simulink model "battery_subsystem"  (R2015a)
settings: Solver=ode23t  StartTime=0.0  StopTime=100  RelTol=1e-3  AbsTol=1e-3
libraries: fl_lib x96
settings Model: CovSFcnEnable=off  Creator=jrivitus  LastModifiedBy=sseshadr
settings OptimizationCC: ExpressionDepthLimit=2147483647
settings DebuggingCC: UnderspecifiedInitializationDetection=Classic  MergeDetectMultiDrivingBlocksExec=none  ParameterPrecisionLossMsg=none  FcnCallInpInsideContextMsg=UseLocalSettings  StateNameClashWarn=warning
settings GRTTargetCC: CombineOutputUpdateFcns=off  GRTInterface=on

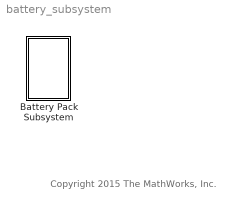
== system battery_subsystem ==
  note: Copyright 2015 The MathWorks, Inc.
  Battery Pack Subsystem : Subsystem

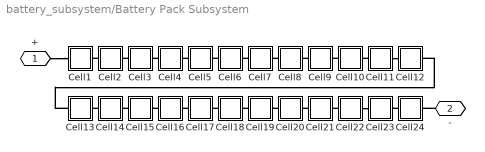
== system battery_subsystem/Battery Pack Subsystem ==
  Cell1 : Subsystem
  Cell10 : Subsystem
  Cell11 : Subsystem
  Cell12 : Subsystem
  Cell13 : Subsystem
  Cell14 : Subsystem
  Cell15 : Subsystem
  Cell16 : Subsystem
  Cell17 : Subsystem
  Cell18 : Subsystem
  Cell19 : Subsystem
  Cell2 : Subsystem
  Cell20 : Subsystem
  Cell21 : Subsystem
  Cell22 : Subsystem
  Cell23 : Subsystem
  Cell24 : Subsystem
  Cell3 : Subsystem
  Cell4 : Subsystem
  Cell5 : Subsystem
  Cell6 : Subsystem
  Cell7 : Subsystem
  Cell8 : Subsystem
  Cell9 : Subsystem
  + : PMIOPort  Port=1  Side=Right
  - : PMIOPort  Port=2  Side=Right
  connections:
  +/RConn1 -- Cell1/LConn1
  Cell2/LConn1 -- Cell1/RConn1
  Cell3/LConn1 -- Cell2/RConn1
  Cell4/LConn1 -- Cell3/RConn1
  Cell5/LConn1 -- Cell4/RConn1
  Cell6/LConn1 -- Cell5/RConn1
  Cell7/LConn1 -- Cell6/RConn1
  Cell8/LConn1 -- Cell7/RConn1
  Cell9/LConn1 -- Cell8/RConn1
  Cell10/LConn1 -- Cell9/RConn1
  Cell11/LConn1 -- Cell10/RConn1
  Cell13/LConn1 -- Cell12/RConn1
  Cell14/LConn1 -- Cell13/RConn1
  Cell15/LConn1 -- Cell14/RConn1
  Cell16/LConn1 -- Cell15/RConn1
  Cell17/LConn1 -- Cell16/RConn1
  Cell18/LConn1 -- Cell17/RConn1
  Cell19/LConn1 -- Cell18/RConn1
  Cell20/LConn1 -- Cell19/RConn1
  Cell21/LConn1 -- Cell20/RConn1
  Cell22/LConn1 -- Cell21/RConn1
  Cell24/LConn1 -- Cell23/RConn1
  -/RConn1 -- Cell24/RConn1
  Cell11/RConn1 -- Cell12/LConn1
  Cell22/RConn1 -- Cell23/LConn1

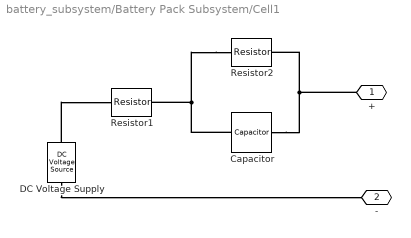
== system battery_subsystem/Battery Pack Subsystem/Cell1 ==
  Capacitor : fl_lib/Electrical/Electrical Elements/Capacitor  c=1e-3 F  r=1e-6 Ohm  g=0 1/Ohm  i_specify=off  i_priority=High  i=0 A  v_specify=off  v_priority=High  v=0 V  vc_specify=on  vc_priority=High  vc=0 V
  DC Voltage Supply : fl_lib/Electrical/Electrical Sources/DC Voltage Source  v0=4.2 V
  Resistor1 : fl_lib/Electrical/Electrical Elements/Resistor  R=0.07 Ohm  i_specify=off  i_priority=High  i=0 A  v_specify=off  v_priority=High  v=0 V
  Resistor2 : fl_lib/Electrical/Electrical Elements/Resistor  R=0.05 Ohm  i_specify=off  i_priority=High  i=0 A  v_specify=off  v_priority=High  v=0 V
  + : PMIOPort  Port=1  Side=Left
  - : PMIOPort  Port=2  Side=Right
  connections:
  Resistor2/LConn1 -- Capacitor/LConn1 -- Resistor1/RConn1
  DC Voltage Supply/RConn1 -- -/RConn1
  Resistor2/RConn1 -- +/RConn1 -- Capacitor/RConn1
  DC Voltage Supply/LConn1 -- Resistor1/LConn1

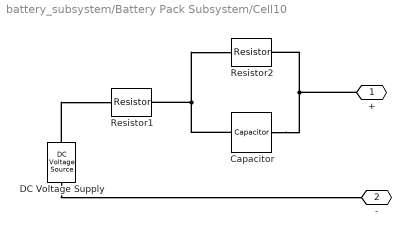
== system battery_subsystem/Battery Pack Subsystem/Cell10 ==
  Capacitor : fl_lib/Electrical/Electrical Elements/Capacitor  c=1e-3 F  r=1e-6 Ohm  g=0 1/Ohm  i_specify=off  i_priority=High  i=0 A  v_specify=off  v_priority=High  v=0 V  vc_specify=on  vc_priority=High  vc=0 V
  DC Voltage Supply : fl_lib/Electrical/Electrical Sources/DC Voltage Source  v0=4.2 V
  Resistor1 : fl_lib/Electrical/Electrical Elements/Resistor  R=0.07 Ohm  i_specify=off  i_priority=High  i=0 A  v_specify=off  v_priority=High  v=0 V
  Resistor2 : fl_lib/Electrical/Electrical Elements/Resistor  R=0.05 Ohm  i_specify=off  i_priority=High  i=0 A  v_specify=off  v_priority=High  v=0 V
  + : PMIOPort  Port=1  Side=Left
  - : PMIOPort  Port=2  Side=Right
  connections:
  DC Voltage Supply/LConn1 -- Resistor1/LConn1
  +/RConn1 -- Capacitor/RConn1 -- Resistor2/RConn1
  DC Voltage Supply/RConn1 -- -/RConn1
  Resistor1/RConn1 -- Capacitor/LConn1 -- Resistor2/LConn1

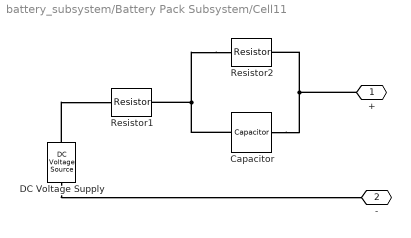
== system battery_subsystem/Battery Pack Subsystem/Cell11 ==
  Capacitor : fl_lib/Electrical/Electrical Elements/Capacitor  c=1e-3 F  r=1e-6 Ohm  g=0 1/Ohm  i_specify=off  i_priority=High  i=0 A  v_specify=off  v_priority=High  v=0 V  vc_specify=on  vc_priority=High  vc=0 V
  DC Voltage Supply : fl_lib/Electrical/Electrical Sources/DC Voltage Source  v0=4.2 V
  Resistor1 : fl_lib/Electrical/Electrical Elements/Resistor  R=0.07 Ohm  i_specify=off  i_priority=High  i=0 A  v_specify=off  v_priority=High  v=0 V
  Resistor2 : fl_lib/Electrical/Electrical Elements/Resistor  R=0.05 Ohm  i_specify=off  i_priority=High  i=0 A  v_specify=off  v_priority=High  v=0 V
  + : PMIOPort  Port=1  Side=Left
  - : PMIOPort  Port=2  Side=Right
  connections:
  Resistor2/LConn1 -- Capacitor/LConn1 -- Resistor1/RConn1
  DC Voltage Supply/RConn1 -- -/RConn1
  Resistor2/RConn1 -- Capacitor/RConn1 -- +/RConn1
  DC Voltage Supply/LConn1 -- Resistor1/LConn1

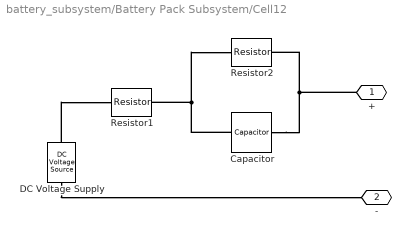
== system battery_subsystem/Battery Pack Subsystem/Cell12 ==
  Capacitor : fl_lib/Electrical/Electrical Elements/Capacitor  c=1e-3 F  r=1e-6 Ohm  g=0 1/Ohm  i_specify=off  i_priority=High  i=0 A  v_specify=off  v_priority=High  v=0 V  vc_specify=on  vc_priority=High  vc=0 V
  DC Voltage Supply : fl_lib/Electrical/Electrical Sources/DC Voltage Source  v0=4.2 V
  Resistor1 : fl_lib/Electrical/Electrical Elements/Resistor  R=0.07 Ohm  i_specify=off  i_priority=High  i=0 A  v_specify=off  v_priority=High  v=0 V
  Resistor2 : fl_lib/Electrical/Electrical Elements/Resistor  R=0.05 Ohm  i_specify=off  i_priority=High  i=0 A  v_specify=off  v_priority=High  v=0 V
  + : PMIOPort  Port=1  Side=Left
  - : PMIOPort  Port=2  Side=Right
  connections:
  DC Voltage Supply/LConn1 -- Resistor1/LConn1
  +/RConn1 -- Capacitor/RConn1 -- Resistor2/RConn1
  DC Voltage Supply/RConn1 -- -/RConn1
  Resistor1/RConn1 -- Capacitor/LConn1 -- Resistor2/LConn1

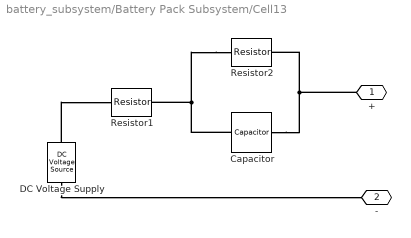
== system battery_subsystem/Battery Pack Subsystem/Cell13 ==
  Capacitor : fl_lib/Electrical/Electrical Elements/Capacitor  c=1e-3 F  r=1e-6 Ohm  g=0 1/Ohm  i_specify=off  i_priority=High  i=0 A  v_specify=off  v_priority=High  v=0 V  vc_specify=on  vc_priority=High  vc=0 V
  DC Voltage Supply : fl_lib/Electrical/Electrical Sources/DC Voltage Source  v0=4.2 V
  Resistor1 : fl_lib/Electrical/Electrical Elements/Resistor  R=0.07 Ohm  i_specify=off  i_priority=High  i=0 A  v_specify=off  v_priority=High  v=0 V
  Resistor2 : fl_lib/Electrical/Electrical Elements/Resistor  R=0.05 Ohm  i_specify=off  i_priority=High  i=0 A  v_specify=off  v_priority=High  v=0 V
  + : PMIOPort  Port=1  Side=Left
  - : PMIOPort  Port=2  Side=Right
  connections:
  Resistor2/LConn1 -- Capacitor/LConn1 -- Resistor1/RConn1
  DC Voltage Supply/RConn1 -- -/RConn1
  Resistor2/RConn1 -- Capacitor/RConn1 -- +/RConn1
  DC Voltage Supply/LConn1 -- Resistor1/LConn1

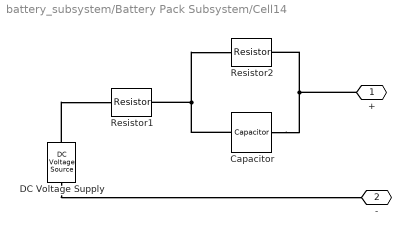
== system battery_subsystem/Battery Pack Subsystem/Cell14 ==
  Capacitor : fl_lib/Electrical/Electrical Elements/Capacitor  c=1e-3 F  r=1e-6 Ohm  g=0 1/Ohm  i_specify=off  i_priority=High  i=0 A  v_specify=off  v_priority=High  v=0 V  vc_specify=on  vc_priority=High  vc=0 V
  DC Voltage Supply : fl_lib/Electrical/Electrical Sources/DC Voltage Source  v0=4.2 V
  Resistor1 : fl_lib/Electrical/Electrical Elements/Resistor  R=0.07 Ohm  i_specify=off  i_priority=High  i=0 A  v_specify=off  v_priority=High  v=0 V
  Resistor2 : fl_lib/Electrical/Electrical Elements/Resistor  R=0.05 Ohm  i_specify=off  i_priority=High  i=0 A  v_specify=off  v_priority=High  v=0 V
  + : PMIOPort  Port=1  Side=Left
  - : PMIOPort  Port=2  Side=Right
  connections:
  DC Voltage Supply/LConn1 -- Resistor1/LConn1
  +/RConn1 -- Capacitor/RConn1 -- Resistor2/RConn1
  DC Voltage Supply/RConn1 -- -/RConn1
  Resistor1/RConn1 -- Capacitor/LConn1 -- Resistor2/LConn1

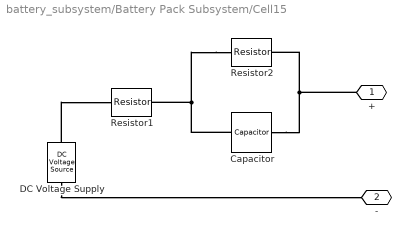
== system battery_subsystem/Battery Pack Subsystem/Cell15 ==
  Capacitor : fl_lib/Electrical/Electrical Elements/Capacitor  c=1e-3 F  r=1e-6 Ohm  g=0 1/Ohm  i_specify=off  i_priority=High  i=0 A  v_specify=off  v_priority=High  v=0 V  vc_specify=on  vc_priority=High  vc=0 V
  DC Voltage Supply : fl_lib/Electrical/Electrical Sources/DC Voltage Source  v0=4.2 V
  Resistor1 : fl_lib/Electrical/Electrical Elements/Resistor  R=0.07 Ohm  i_specify=off  i_priority=High  i=0 A  v_specify=off  v_priority=High  v=0 V
  Resistor2 : fl_lib/Electrical/Electrical Elements/Resistor  R=0.05 Ohm  i_specify=off  i_priority=High  i=0 A  v_specify=off  v_priority=High  v=0 V
  + : PMIOPort  Port=1  Side=Left
  - : PMIOPort  Port=2  Side=Right
  connections:
  Resistor2/LConn1 -- Capacitor/LConn1 -- Resistor1/RConn1
  DC Voltage Supply/RConn1 -- -/RConn1
  Resistor2/RConn1 -- Capacitor/RConn1 -- +/RConn1
  DC Voltage Supply/LConn1 -- Resistor1/LConn1

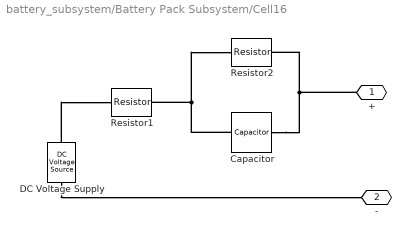
== system battery_subsystem/Battery Pack Subsystem/Cell16 ==
  Capacitor : fl_lib/Electrical/Electrical Elements/Capacitor  c=1e-3 F  r=1e-6 Ohm  g=0 1/Ohm  i_specify=off  i_priority=High  i=0 A  v_specify=off  v_priority=High  v=0 V  vc_specify=on  vc_priority=High  vc=0 V
  DC Voltage Supply : fl_lib/Electrical/Electrical Sources/DC Voltage Source  v0=4.2 V
  Resistor1 : fl_lib/Electrical/Electrical Elements/Resistor  R=0.07 Ohm  i_specify=off  i_priority=High  i=0 A  v_specify=off  v_priority=High  v=0 V
  Resistor2 : fl_lib/Electrical/Electrical Elements/Resistor  R=0.05 Ohm  i_specify=off  i_priority=High  i=0 A  v_specify=off  v_priority=High  v=0 V
  + : PMIOPort  Port=1  Side=Left
  - : PMIOPort  Port=2  Side=Right
  connections:
  DC Voltage Supply/LConn1 -- Resistor1/LConn1
  +/RConn1 -- Capacitor/RConn1 -- Resistor2/RConn1
  DC Voltage Supply/RConn1 -- -/RConn1
  Resistor1/RConn1 -- Capacitor/LConn1 -- Resistor2/LConn1

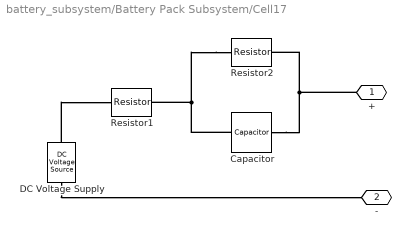
== system battery_subsystem/Battery Pack Subsystem/Cell17 ==
  Capacitor : fl_lib/Electrical/Electrical Elements/Capacitor  c=1e-3 F  r=1e-6 Ohm  g=0 1/Ohm  i_specify=off  i_priority=High  i=0 A  v_specify=off  v_priority=High  v=0 V  vc_specify=on  vc_priority=High  vc=0 V
  DC Voltage Supply : fl_lib/Electrical/Electrical Sources/DC Voltage Source  v0=4.2 V
  Resistor1 : fl_lib/Electrical/Electrical Elements/Resistor  R=0.07 Ohm  i_specify=off  i_priority=High  i=0 A  v_specify=off  v_priority=High  v=0 V
  Resistor2 : fl_lib/Electrical/Electrical Elements/Resistor  R=0.05 Ohm  i_specify=off  i_priority=High  i=0 A  v_specify=off  v_priority=High  v=0 V
  + : PMIOPort  Port=1  Side=Left
  - : PMIOPort  Port=2  Side=Right
  connections:
  Resistor2/LConn1 -- Capacitor/LConn1 -- Resistor1/RConn1
  DC Voltage Supply/RConn1 -- -/RConn1
  Resistor2/RConn1 -- Capacitor/RConn1 -- +/RConn1
  DC Voltage Supply/LConn1 -- Resistor1/LConn1

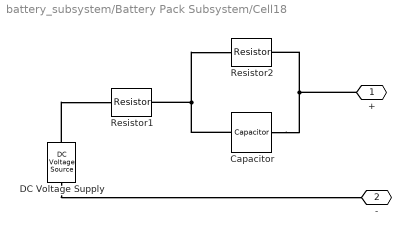
== system battery_subsystem/Battery Pack Subsystem/Cell18 ==
  Capacitor : fl_lib/Electrical/Electrical Elements/Capacitor  c=1e-3 F  r=1e-6 Ohm  g=0 1/Ohm  i_specify=off  i_priority=High  i=0 A  v_specify=off  v_priority=High  v=0 V  vc_specify=on  vc_priority=High  vc=0 V
  DC Voltage Supply : fl_lib/Electrical/Electrical Sources/DC Voltage Source  v0=4.2 V
  Resistor1 : fl_lib/Electrical/Electrical Elements/Resistor  R=0.07 Ohm  i_specify=off  i_priority=High  i=0 A  v_specify=off  v_priority=High  v=0 V
  Resistor2 : fl_lib/Electrical/Electrical Elements/Resistor  R=0.05 Ohm  i_specify=off  i_priority=High  i=0 A  v_specify=off  v_priority=High  v=0 V
  + : PMIOPort  Port=1  Side=Left
  - : PMIOPort  Port=2  Side=Right
  connections:
  DC Voltage Supply/LConn1 -- Resistor1/LConn1
  +/RConn1 -- Capacitor/RConn1 -- Resistor2/RConn1
  DC Voltage Supply/RConn1 -- -/RConn1
  Resistor1/RConn1 -- Capacitor/LConn1 -- Resistor2/LConn1

== system battery_subsystem/Battery Pack Subsystem/Cell19 ==
  Capacitor : fl_lib/Electrical/Electrical Elements/Capacitor  c=1e-3 F  r=1e-6 Ohm  g=0 1/Ohm  i_specify=off  i_priority=High  i=0 A  v_specify=off  v_priority=High  v=0 V  vc_specify=on  vc_priority=High  vc=0 V
  DC Voltage Supply : fl_lib/Electrical/Electrical Sources/DC Voltage Source  v0=4.2 V
  Resistor1 : fl_lib/Electrical/Electrical Elements/Resistor  R=0.07 Ohm  i_specify=off  i_priority=High  i=0 A  v_specify=off  v_priority=High  v=0 V
  Resistor2 : fl_lib/Electrical/Electrical Elements/Resistor  R=0.05 Ohm  i_specify=off  i_priority=High  i=0 A  v_specify=off  v_priority=High  v=0 V
  + : PMIOPort  Port=1  Side=Left
  - : PMIOPort  Port=2  Side=Right
  connections:
  Resistor2/LConn1 -- Capacitor/LConn1 -- Resistor1/RConn1
  DC Voltage Supply/RConn1 -- -/RConn1
  Resistor2/RConn1 -- Capacitor/RConn1 -- +/RConn1
  DC Voltage Supply/LConn1 -- Resistor1/LConn1

== system battery_subsystem/Battery Pack Subsystem/Cell2 ==
  Capacitor : fl_lib/Electrical/Electrical Elements/Capacitor  c=1e-3 F  r=1e-6 Ohm  g=0 1/Ohm  i_specify=off  i_priority=High  i=0 A  v_specify=off  v_priority=High  v=0 V  vc_specify=on  vc_priority=High  vc=0 V
  DC Voltage Supply : fl_lib/Electrical/Electrical Sources/DC Voltage Source  v0=4.2 V
  Resistor1 : fl_lib/Electrical/Electrical Elements/Resistor  R=0.07 Ohm  i_specify=off  i_priority=High  i=0 A  v_specify=off  v_priority=High  v=0 V
  Resistor2 : fl_lib/Electrical/Electrical Elements/Resistor  R=0.05 Ohm  i_specify=off  i_priority=High  i=0 A  v_specify=off  v_priority=High  v=0 V
  + : PMIOPort  Port=1  Side=Left
  - : PMIOPort  Port=2  Side=Right
  connections:
  DC Voltage Supply/LConn1 -- Resistor1/LConn1
  +/RConn1 -- Capacitor/RConn1 -- Resistor2/RConn1
  DC Voltage Supply/RConn1 -- -/RConn1
  Resistor1/RConn1 -- Capacitor/LConn1 -- Resistor2/LConn1

== system battery_subsystem/Battery Pack Subsystem/Cell20 ==
  Capacitor : fl_lib/Electrical/Electrical Elements/Capacitor  c=1e-3 F  r=1e-6 Ohm  g=0 1/Ohm  i_specify=off  i_priority=High  i=0 A  v_specify=off  v_priority=High  v=0 V  vc_specify=on  vc_priority=High  vc=0 V
  DC Voltage Supply : fl_lib/Electrical/Electrical Sources/DC Voltage Source  v0=4.2 V
  Resistor1 : fl_lib/Electrical/Electrical Elements/Resistor  R=0.07 Ohm  i_specify=off  i_priority=High  i=0 A  v_specify=off  v_priority=High  v=0 V
  Resistor2 : fl_lib/Electrical/Electrical Elements/Resistor  R=0.05 Ohm  i_specify=off  i_priority=High  i=0 A  v_specify=off  v_priority=High  v=0 V
  + : PMIOPort  Port=1  Side=Left
  - : PMIOPort  Port=2  Side=Right
  connections:
  DC Voltage Supply/LConn1 -- Resistor1/LConn1
  +/RConn1 -- Capacitor/RConn1 -- Resistor2/RConn1
  DC Voltage Supply/RConn1 -- -/RConn1
  Resistor1/RConn1 -- Capacitor/LConn1 -- Resistor2/LConn1

== system battery_subsystem/Battery Pack Subsystem/Cell21 ==
  Capacitor : fl_lib/Electrical/Electrical Elements/Capacitor  c=1e-3 F  r=1e-6 Ohm  g=0 1/Ohm  i_specify=off  i_priority=High  i=0 A  v_specify=off  v_priority=High  v=0 V  vc_specify=on  vc_priority=High  vc=0 V
  DC Voltage Supply : fl_lib/Electrical/Electrical Sources/DC Voltage Source  v0=4.2 V
  Resistor1 : fl_lib/Electrical/Electrical Elements/Resistor  R=0.07 Ohm  i_specify=off  i_priority=High  i=0 A  v_specify=off  v_priority=High  v=0 V
  Resistor2 : fl_lib/Electrical/Electrical Elements/Resistor  R=0.05 Ohm  i_specify=off  i_priority=High  i=0 A  v_specify=off  v_priority=High  v=0 V
  + : PMIOPort  Port=1  Side=Left
  - : PMIOPort  Port=2  Side=Right
  connections:
  Resistor2/LConn1 -- Capacitor/LConn1 -- Resistor1/RConn1
  DC Voltage Supply/RConn1 -- -/RConn1
  Resistor2/RConn1 -- Capacitor/RConn1 -- +/RConn1
  DC Voltage Supply/LConn1 -- Resistor1/LConn1

== system battery_subsystem/Battery Pack Subsystem/Cell22 ==
  Capacitor : fl_lib/Electrical/Electrical Elements/Capacitor  c=1e-3 F  r=1e-6 Ohm  g=0 1/Ohm  i_specify=off  i_priority=High  i=0 A  v_specify=off  v_priority=High  v=0 V  vc_specify=on  vc_priority=High  vc=0 V
  DC Voltage Supply : fl_lib/Electrical/Electrical Sources/DC Voltage Source  v0=4.2 V
  Resistor1 : fl_lib/Electrical/Electrical Elements/Resistor  R=0.07 Ohm  i_specify=off  i_priority=High  i=0 A  v_specify=off  v_priority=High  v=0 V
  Resistor2 : fl_lib/Electrical/Electrical Elements/Resistor  R=0.05 Ohm  i_specify=off  i_priority=High  i=0 A  v_specify=off  v_priority=High  v=0 V
  + : PMIOPort  Port=1  Side=Left
  - : PMIOPort  Port=2  Side=Right
  connections:
  DC Voltage Supply/LConn1 -- Resistor1/LConn1
  +/RConn1 -- Capacitor/RConn1 -- Resistor2/RConn1
  DC Voltage Supply/RConn1 -- -/RConn1
  Resistor1/RConn1 -- Capacitor/LConn1 -- Resistor2/LConn1

== system battery_subsystem/Battery Pack Subsystem/Cell23 ==
  Capacitor : fl_lib/Electrical/Electrical Elements/Capacitor  c=1e-3 F  r=1e-6 Ohm  g=0 1/Ohm  i_specify=off  i_priority=High  i=0 A  v_specify=off  v_priority=High  v=0 V  vc_specify=on  vc_priority=High  vc=0 V
  DC Voltage Supply : fl_lib/Electrical/Electrical Sources/DC Voltage Source  v0=4.2 V
  Resistor1 : fl_lib/Electrical/Electrical Elements/Resistor  R=0.07 Ohm  i_specify=off  i_priority=High  i=0 A  v_specify=off  v_priority=High  v=0 V
  Resistor2 : fl_lib/Electrical/Electrical Elements/Resistor  R=0.05 Ohm  i_specify=off  i_priority=High  i=0 A  v_specify=off  v_priority=High  v=0 V
  + : PMIOPort  Port=1  Side=Left
  - : PMIOPort  Port=2  Side=Right
  connections:
  Resistor2/LConn1 -- Capacitor/LConn1 -- Resistor1/RConn1
  DC Voltage Supply/RConn1 -- -/RConn1
  Resistor2/RConn1 -- Capacitor/RConn1 -- +/RConn1
  DC Voltage Supply/LConn1 -- Resistor1/LConn1

== system battery_subsystem/Battery Pack Subsystem/Cell24 ==
  Capacitor : fl_lib/Electrical/Electrical Elements/Capacitor  c=1e-3 F  r=1e-6 Ohm  g=0 1/Ohm  i_specify=off  i_priority=High  i=0 A  v_specify=off  v_priority=High  v=0 V  vc_specify=on  vc_priority=High  vc=0 V
  DC Voltage Supply : fl_lib/Electrical/Electrical Sources/DC Voltage Source  v0=4.2 V
  Resistor1 : fl_lib/Electrical/Electrical Elements/Resistor  R=0.07 Ohm  i_specify=off  i_priority=High  i=0 A  v_specify=off  v_priority=High  v=0 V
  Resistor2 : fl_lib/Electrical/Electrical Elements/Resistor  R=0.05 Ohm  i_specify=off  i_priority=High  i=0 A  v_specify=off  v_priority=High  v=0 V
  + : PMIOPort  Port=1  Side=Left
  - : PMIOPort  Port=2  Side=Right
  connections:
  DC Voltage Supply/LConn1 -- Resistor1/LConn1
  +/RConn1 -- Capacitor/RConn1 -- Resistor2/RConn1
  DC Voltage Supply/RConn1 -- -/RConn1
  Resistor1/RConn1 -- Capacitor/LConn1 -- Resistor2/LConn1

== system battery_subsystem/Battery Pack Subsystem/Cell3 ==
  Capacitor : fl_lib/Electrical/Electrical Elements/Capacitor  c=1e-3 F  r=1e-6 Ohm  g=0 1/Ohm  i_specify=off  i_priority=High  i=0 A  v_specify=off  v_priority=High  v=0 V  vc_specify=on  vc_priority=High  vc=0 V
  DC Voltage Supply : fl_lib/Electrical/Electrical Sources/DC Voltage Source  v0=4.2 V
  Resistor1 : fl_lib/Electrical/Electrical Elements/Resistor  R=0.07 Ohm  i_specify=off  i_priority=High  i=0 A  v_specify=off  v_priority=High  v=0 V
  Resistor2 : fl_lib/Electrical/Electrical Elements/Resistor  R=0.05 Ohm  i_specify=off  i_priority=High  i=0 A  v_specify=off  v_priority=High  v=0 V
  + : PMIOPort  Port=1  Side=Left
  - : PMIOPort  Port=2  Side=Right
  connections:
  Resistor2/LConn1 -- Capacitor/LConn1 -- Resistor1/RConn1
  DC Voltage Supply/RConn1 -- -/RConn1
  Resistor2/RConn1 -- Capacitor/RConn1 -- +/RConn1
  DC Voltage Supply/LConn1 -- Resistor1/LConn1

== system battery_subsystem/Battery Pack Subsystem/Cell4 ==
  Capacitor : fl_lib/Electrical/Electrical Elements/Capacitor  c=1e-3 F  r=1e-6 Ohm  g=0 1/Ohm  i_specify=off  i_priority=High  i=0 A  v_specify=off  v_priority=High  v=0 V  vc_specify=on  vc_priority=High  vc=0 V
  DC Voltage Supply : fl_lib/Electrical/Electrical Sources/DC Voltage Source  v0=4.2 V
  Resistor1 : fl_lib/Electrical/Electrical Elements/Resistor  R=0.07 Ohm  i_specify=off  i_priority=High  i=0 A  v_specify=off  v_priority=High  v=0 V
  Resistor2 : fl_lib/Electrical/Electrical Elements/Resistor  R=0.05 Ohm  i_specify=off  i_priority=High  i=0 A  v_specify=off  v_priority=High  v=0 V
  + : PMIOPort  Port=1  Side=Left
  - : PMIOPort  Port=2  Side=Right
  connections:
  DC Voltage Supply/LConn1 -- Resistor1/LConn1
  +/RConn1 -- Capacitor/RConn1 -- Resistor2/RConn1
  DC Voltage Supply/RConn1 -- -/RConn1
  Resistor1/RConn1 -- Capacitor/LConn1 -- Resistor2/LConn1

== system battery_subsystem/Battery Pack Subsystem/Cell5 ==
  Capacitor : fl_lib/Electrical/Electrical Elements/Capacitor  c=1e-3 F  r=1e-6 Ohm  g=0 1/Ohm  i_specify=off  i_priority=High  i=0 A  v_specify=off  v_priority=High  v=0 V  vc_specify=on  vc_priority=High  vc=0 V
  DC Voltage Supply : fl_lib/Electrical/Electrical Sources/DC Voltage Source  v0=4.2 V
  Resistor1 : fl_lib/Electrical/Electrical Elements/Resistor  R=0.07 Ohm  i_specify=off  i_priority=High  i=0 A  v_specify=off  v_priority=High  v=0 V
  Resistor2 : fl_lib/Electrical/Electrical Elements/Resistor  R=0.05 Ohm  i_specify=off  i_priority=High  i=0 A  v_specify=off  v_priority=High  v=0 V
  + : PMIOPort  Port=1  Side=Left
  - : PMIOPort  Port=2  Side=Right
  connections:
  Resistor2/LConn1 -- Capacitor/LConn1 -- Resistor1/RConn1
  DC Voltage Supply/RConn1 -- -/RConn1
  Resistor2/RConn1 -- Capacitor/RConn1 -- +/RConn1
  DC Voltage Supply/LConn1 -- Resistor1/LConn1

== system battery_subsystem/Battery Pack Subsystem/Cell6 ==
  Capacitor : fl_lib/Electrical/Electrical Elements/Capacitor  c=1e-3 F  r=1e-6 Ohm  g=0 1/Ohm  i_specify=off  i_priority=High  i=0 A  v_specify=off  v_priority=High  v=0 V  vc_specify=on  vc_priority=High  vc=0 V
  DC Voltage Supply : fl_lib/Electrical/Electrical Sources/DC Voltage Source  v0=4.2 V
  Resistor1 : fl_lib/Electrical/Electrical Elements/Resistor  R=0.07 Ohm  i_specify=off  i_priority=High  i=0 A  v_specify=off  v_priority=High  v=0 V
  Resistor2 : fl_lib/Electrical/Electrical Elements/Resistor  R=0.05 Ohm  i_specify=off  i_priority=High  i=0 A  v_specify=off  v_priority=High  v=0 V
  + : PMIOPort  Port=1  Side=Left
  - : PMIOPort  Port=2  Side=Right
  connections:
  DC Voltage Supply/LConn1 -- Resistor1/LConn1
  +/RConn1 -- Capacitor/RConn1 -- Resistor2/RConn1
  DC Voltage Supply/RConn1 -- -/RConn1
  Resistor1/RConn1 -- Capacitor/LConn1 -- Resistor2/LConn1

== system battery_subsystem/Battery Pack Subsystem/Cell7 ==
  Capacitor : fl_lib/Electrical/Electrical Elements/Capacitor  c=1e-3 F  r=1e-6 Ohm  g=0 1/Ohm  i_specify=off  i_priority=High  i=0 A  v_specify=off  v_priority=High  v=0 V  vc_specify=on  vc_priority=High  vc=0 V
  DC Voltage Supply : fl_lib/Electrical/Electrical Sources/DC Voltage Source  v0=4.2 V
  Resistor1 : fl_lib/Electrical/Electrical Elements/Resistor  R=0.07 Ohm  i_specify=off  i_priority=High  i=0 A  v_specify=off  v_priority=High  v=0 V
  Resistor2 : fl_lib/Electrical/Electrical Elements/Resistor  R=0.05 Ohm  i_specify=off  i_priority=High  i=0 A  v_specify=off  v_priority=High  v=0 V
  + : PMIOPort  Port=1  Side=Left
  - : PMIOPort  Port=2  Side=Right
  connections:
  Resistor2/LConn1 -- Capacitor/LConn1 -- Resistor1/RConn1
  DC Voltage Supply/RConn1 -- -/RConn1
  Resistor2/RConn1 -- Capacitor/RConn1 -- +/RConn1
  DC Voltage Supply/LConn1 -- Resistor1/LConn1

== system battery_subsystem/Battery Pack Subsystem/Cell8 ==
  Capacitor : fl_lib/Electrical/Electrical Elements/Capacitor  c=1e-3 F  r=1e-6 Ohm  g=0 1/Ohm  i_specify=off  i_priority=High  i=0 A  v_specify=off  v_priority=High  v=0 V  vc_specify=on  vc_priority=High  vc=0 V
  DC Voltage Supply : fl_lib/Electrical/Electrical Sources/DC Voltage Source  v0=4.2 V
  Resistor1 : fl_lib/Electrical/Electrical Elements/Resistor  R=0.07 Ohm  i_specify=off  i_priority=High  i=0 A  v_specify=off  v_priority=High  v=0 V
  Resistor2 : fl_lib/Electrical/Electrical Elements/Resistor  R=0.05 Ohm  i_specify=off  i_priority=High  i=0 A  v_specify=off  v_priority=High  v=0 V
  + : PMIOPort  Port=1  Side=Left
  - : PMIOPort  Port=2  Side=Right
  connections:
  DC Voltage Supply/LConn1 -- Resistor1/LConn1
  +/RConn1 -- Capacitor/RConn1 -- Resistor2/RConn1
  DC Voltage Supply/RConn1 -- -/RConn1
  Resistor1/RConn1 -- Capacitor/LConn1 -- Resistor2/LConn1

== system battery_subsystem/Battery Pack Subsystem/Cell9 ==
  Capacitor : fl_lib/Electrical/Electrical Elements/Capacitor  c=1e-3 F  r=1e-6 Ohm  g=0 1/Ohm  i_specify=off  i_priority=High  i=0 A  v_specify=off  v_priority=High  v=0 V  vc_specify=on  vc_priority=High  vc=0 V
  DC Voltage Supply : fl_lib/Electrical/Electrical Sources/DC Voltage Source  v0=4.2 V
  Resistor1 : fl_lib/Electrical/Electrical Elements/Resistor  R=0.07 Ohm  i_specify=off  i_priority=High  i=0 A  v_specify=off  v_priority=High  v=0 V
  Resistor2 : fl_lib/Electrical/Electrical Elements/Resistor  R=0.05 Ohm  i_specify=off  i_priority=High  i=0 A  v_specify=off  v_priority=High  v=0 V
  + : PMIOPort  Port=1  Side=Left
  - : PMIOPort  Port=2  Side=Right
  connections:
  Resistor2/LConn1 -- Capacitor/LConn1 -- Resistor1/RConn1
  DC Voltage Supply/RConn1 -- -/RConn1
  Resistor2/RConn1 -- Capacitor/RConn1 -- +/RConn1
  DC Voltage Supply/LConn1 -- Resistor1/LConn1
